simulink subsystem "StatePropagation"  (R2022a)
settings: Solver=VariableStepAuto  StartTime=0.0  StopTime=10.0  RelTol=1e-3
model mask{spaceRobot=spaceRobot, jointCstr=on, q_0=0, q_dot_0=0}
  mask prompts: jointCstr "Apply joint constraints?"; q_0 "Config"; q_dot_0 "Speed"
undefined symbols (not defined in the file): jointLims
settings Model: Creator=charl  LastModifiedBy=charl

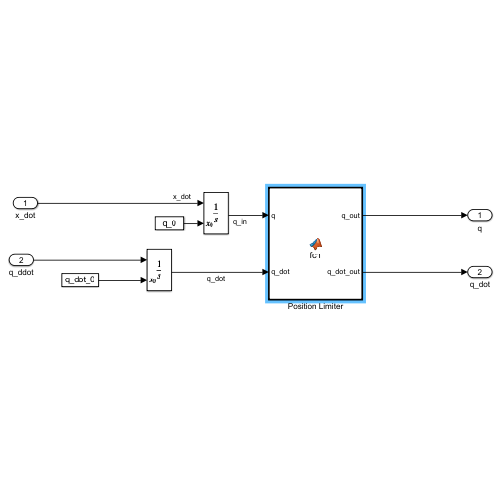
[thumbnail: Simulink's stored preview of the top-level diagram]
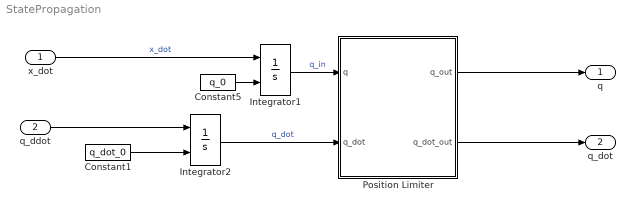
== system StatePropagation ==
  x_dot : Inport
  q_ddot : Inport  Port=2
  Constant1 : Constant  Value=q_dot_0
  Constant5 : Constant  Value=q_0
  Integrator1 : Integrator  InitialConditionSource=external
  Integrator2 : Integrator  InitialConditionSource=external
  Position Limiter : MATLAB Function  TreatAsAtomicUnit=on
  q : Outport
  q_dot : Outport  Port=2
  wires:
  x_dot/1 -> Integrator1/1  "x_dot"
  Integrator1/1 -> Position Limiter/1(q)  "q_in"
  Constant5/1 -> Integrator1/2
  Position Limiter/1(q_out) -> q/1
  Position Limiter/2(q_dot_out) -> q_dot/1
  Integrator2/1 -> Position Limiter/2(q_dot)  "q_dot"
  Constant1/1 -> Integrator2/2
  q_ddot/1 -> Integrator2/1

== matlab function StatePropagation/Position Limiter ==
  data: q input; q_out output; q_dot input; q_dot_out output; jointLims parameter; jointCstr parameter
function [q_out, q_dot_out] = fcn(q, q_dot, jointLims, jointCstr)

q_out = q;  
q_dot_out = q_dot;

if jointCstr
    for i=7:6+size(jointLims, 1)
        lims = jointLims(i-6, :);
    
    
        if q(i) < lims(1)
            q_out(i) = lims(1);
            q_dot_out(i) = 0;
    
        elseif q(i) > lims(2)
            q_out(i) = lims(2);
            q_dot_out(i) = 0;
        end
    end
end
